simulink model "compensated_system"  (R2023a)
settings: Solver=VariableStepAuto  StartTime=0.0  StopTime=2  RelTol=1e-3
libraries: spsCurrentMeasurementLib x3, spsMeanLib x3, spsSeriesRLCBranchLib x2, spsDCVoltageSourceLib x1, spsDiodeLib x1, spsLinearTransformerLib x1, spsMosfetLib x1, dspstat3 x1, spsSawtoothGeneratorLib x1, spsVoltageMeasurementLib x1, sps_lib x1
settings Model: Creator=anike  LastModifiedBy=anike

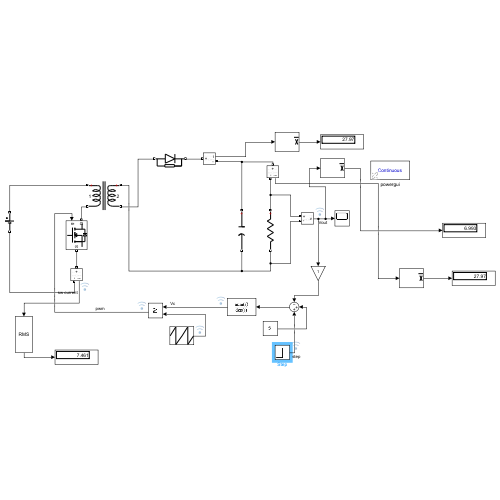
[thumbnail: Simulink's stored preview of the top-level diagram]
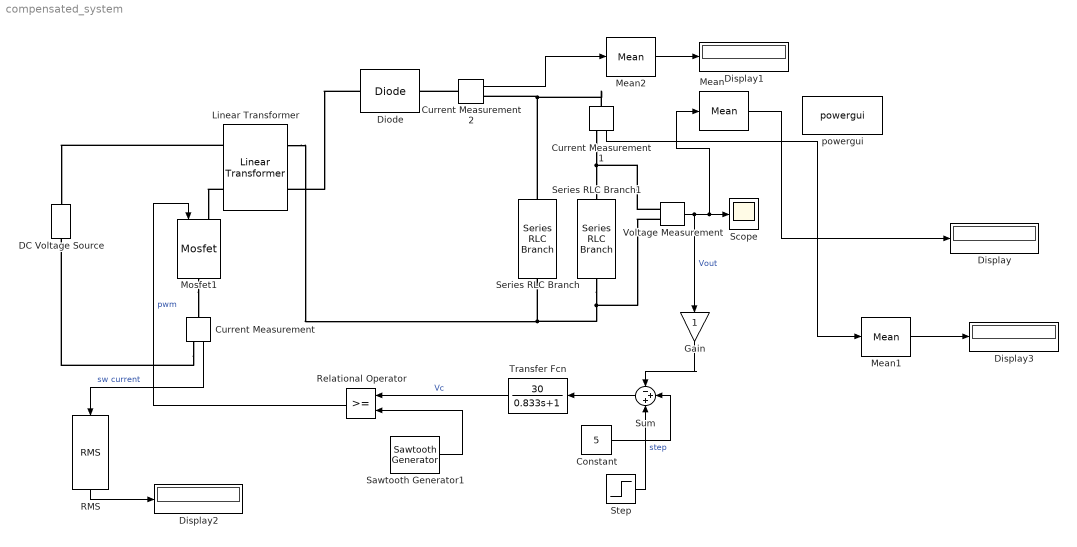
== system compensated_system ==
  Constant : Constant  Value=5
  Current Measurement : spsCurrentMeasurementLib/Current Measurement  PhasorSimulation=off  OutputType=Complex  PSBequivalent=0
  Current Measurement1 : spsCurrentMeasurementLib/Current Measurement  PhasorSimulation=off  OutputType=Complex  PSBequivalent=0
  Current Measurement2 : spsCurrentMeasurementLib/Current Measurement  PhasorSimulation=off  OutputType=Complex  PSBequivalent=0
  DC Voltage Source : spsDCVoltageSourceLib/DC Voltage Source  Amplitude=48  Measurements=None
  Diode : spsDiodeLib/Diode  Ron=0.001  Lon=0  Vf=0.38  IC=0  UseSnubber=0  Rs=500  Cs=250e-9  Measurements=off
  Display{,1..3} (4 alike) : Display
  Gain : Gain
  Linear Transformer : spsLinearTransformerLib/Linear Transformer  UNITS=SI  NominalPower=[ 100 50e3 ]  winding1=[48 0 0]  winding2=[5 0 0]  ThreeWindings=off  winding3=[3.15e+05 0.7938 0.084225]  RmLm=[1.0804e+6 1.360e-3]  Measurements=None  DataType=on
  Mean : spsMeanLib/Mean  Freq=50  Vinit=0  Ts=0
  Mean1 : spsMeanLib/Mean  Freq=50  Vinit=0  Ts=0
  Mean2 : spsMeanLib/Mean  Freq=50  Vinit=0  Ts=0
  Mosfet1 : spsMosfetLib/Mosfet  Ron=0.1  Lon=0  Rd=0.01  Vfd=0  IC=0  Rs=1e5  Cs=inf  Measurements=off
  RMS : dspstat3/RMS  run=off  directionMode=Each column  dimension=1  InputProcessing=Columns as channels (frame based)  reset_popup=None
  Relational Operator : RelationalOperator  OutDataTypeStr=boolean  RndMeth=Simplest  InputSameDT=off
  Sawtooth Generator1 : spsSawtoothGeneratorLib/Sawtooth Generator  Freq=50e3  Phase=180  Ts=0
  Scope : Scope
  Series RLC Branch : spsSeriesRLCBranchLib/Series RLC Branch  LConnTagsString=__new0  RConnTagsString=__new0  BranchType=C  Resistance=1  Inductance=1e-3  SetiL0=off  InitialCurrent=0  Capacitance=3.072e-3  Setx0=off  InitialVoltage=0  Measurements=None
  Series RLC Branch1 : spsSeriesRLCBranchLib/Series RLC Branch  LConnTagsString=__new0  RConnTagsString=__new0  BranchType=R  Resistance=0.25  Inductance=1e-3  SetiL0=off  InitialCurrent=0  Capacitance=3.85e-3  Setx0=off  InitialVoltage=0  Measurements=None
  Step : Step  After=2  SampleTime=0.5
  Sum : Sum  Inputs=-++
  Transfer Fcn : TransferFcn  Numerator=[30]  Denominator=[0.833 1]
  Voltage Measurement : spsVoltageMeasurementLib/Voltage Measurement  PhasorSimulation=off  OutputType=Complex  PSBequivalent=0
  powergui : sps_lib/powergui  Priority=1  SimulationMode=Continuous  SampleTime=50e-6  frequency=60  Iterations=50  frequencyindice=0  Pbase=100e6  ErrMax=1e-4  UnitsV=kV  UnitsW=MW  buscounter=0  FunctionMessages=off  echomessages=off  EnableUseOfTLC=off  CurrentSourceSwitches=off  DisableSnubberDevices=off  DisableRonSwitches=off  DisableVfSwitches=off  DisplayEquations=off  AutomaticDiscreteSolvers=off  SolverType=Tustin/Backward Euler (TBE)  Interpol=off  ExternalGateDelay=off  methode=off  Ts=100  x0status=blocks  SPID=on  SwTol=0  HookPort=off  NonlinearTolerance=1e-4  nMaxIteration=100  ContinueOnMaxIteration=off  RestoreLinks=warning  ResistiveCurrentMeasurement=off  Frange=[0:2:500]  Ylog=off  Xlog=on  ShowGrid=off  save=off  variable=ZData  structure=0  ZoomFFT=off  StartTime=0.0  cycles=1  DisplayStyle=1  fundamental=60  FreqAxis=off  MaxFrequency=1000  frequencyindicesteady=1  RmsSteady=1  display=off
  wires:
  Mean/1 -> Display/1
  Voltage Measurement/1 -> Mean/1, Scope/1, Gain/1  "Vout"
  Relational Operator/1 -> Mosfet1/1  "pwm"
  Sum/1 -> Transfer Fcn/1
  Constant/1 -> Sum/2
  Sawtooth Generator1/1 -> Relational Operator/2
  Transfer Fcn/1 -> Relational Operator/1  "Vc"
  Gain/1 -> Sum/1
  Current Measurement2/1 -> Mean2/1
  Current Measurement1/1 -> Mean1/1
  Mean1/1 -> Display3/1
  Mean2/1 -> Display1/1
  Current Measurement/1 -> RMS/1  "sw current"
  RMS/1 -> Display2/1
  Step/1 -> Sum/3  "step"
  connections:
  Series RLC Branch1/RConn1 -- Voltage Measurement/LConn2 -- Linear Transformer/RConn1 -- Series RLC Branch/RConn1
  Series RLC Branch/LConn1 -- Current Measurement1/LConn1 -- Current Measurement2/RConn1
  Linear Transformer/LConn1 -- DC Voltage Source/RConn1
  Linear Transformer/LConn2 -- Mosfet1/LConn1
  Diode/LConn1 -- Linear Transformer/RConn2
  Current Measurement2/LConn1 -- Diode/RConn1
  Voltage Measurement/LConn1 -- Series RLC Branch1/LConn1 -- Current Measurement1/RConn1
  Mosfet1/RConn1 -- Current Measurement/LConn1
  Current Measurement/RConn1 -- DC Voltage Source/LConn1
